simulink model "rtds_opal_aurora_synchronized"  (Simulink 10.0)
settings: Solver=ode4  StartTime=0.0  StopTime=inf  FixedStep=0.00005  RelTol=1e-3  EnableMultiTasking=on
PreLoadFcn:
  | Ts=50e-6;
InitFcn:
  | Ts=50e-6;
undefined symbols (not defined in the file): DUALSFP, EX, VC707_2
libraries: rtio_opalrt_common x8, rtlab x6, powerlib x6, simulink x3, xpcutilitieslib x1
Description:
  | Model of a simple control system for use iin training.
settings Model: Creator=Paul Baracos  LastModifiedBy=nei
settings Model: SuppressorTable=|
  | <?xml version="1.0" encoding="UTF-8" standalone="yes" ?>
  | <!DOCTYPE boost_serialization>
  | <boost_serialization signature="serialization::archive" version="15">
  | <DiagnosticSuppressor class_id="0" tracking_level="0" version="6">
  | 	<Table class_id="1" tracking_level="0" version="0">
  | 		<count>3</count>
  | 		<bucket_count>8</bucket_count>
  | 		<item_version>0</item_version>
  | 		<item class_id="2" tracking_level="0" version="0">
  | 			<first class_id="3" tracking_level="0" version="6">
  | 				<Source class_id="4" tracking_level="0" version="0">
  | 					<count>1</count>
  | 					<item_version>0</item_version>
  | 					<item>rtds_opal_aurora_synchronized/SM_Controller/Subsystem/Extract Bits</item>
  | 				</Source>
  | 			</first>
  | 			<second class_id="5" tracking_level="0" version="6">
  | 				<SuppressedData class_id="6" tracking_level="0" version="0">
  | 					<count>2</count>
  | 					<bucket_count>8</bucket_count>
  | 					<item_version>0</item_version>
  | 					<item class_id="7" tracking_level="0" version="0">
  | 						<first class_id="8" tracking_level="0" version="6">
  | 							<ID>Simulink:DataType:WarningOverFlowDetected</ID>
  | 							<Cause>
  | 								<Source>
  | 									<count>0</count>
  | 									<item_version>0</item_version>
  | 								</Source>
  | 							</Cause>
  | 						</first>
  | 						<second class_id="9" tracking_level="0" version="6">
  | 							<Comment></Comment>
  | 							<User></User>
  | 							<LastModified class_id="10" tracking_level="0" version="0">
  | 								<ptime_date class_id="11" tracking_level="0" version="0">
  | 									<date>20160608</date>
  | 								</ptime_date>
  | 								<ptime_time_duration class_id="12" tracking_level="0" version="0">
  | 									<is_special>0</is_special>
  | 									<time_duration_hours>15</time_duration_hours>
  | 									<time_duration_minutes>43</time_duration_minutes>
  | 									<time_duration_seconds>6</time_duration_seconds>
  | 									<time_duration_fractional_seconds>0</time_duration_fractional_seconds>
  | 								</ptime_time_duration>
  | 							</LastModified>
  | 							<SuppressionType>1</SuppressionType>
  | 						</second>
  | 					</item>
  | 					<item>
  | 						<first>
  | 							<ID>SimulinkFixedPoint:util:Overflowoccurred</ID>
  | 							<Cause>
  | 								<Source>
  | 									<count>0</count>
  | 									<item_version>0</item_version>
  | 								</Source>
  | 							</Cause>
  | 						</first>
  | 						<second>
  | 							<Comment></Comment>
  | 							<User></User>
  | 							<LastModified>
  | 								<ptime_date>
  | 									<date>20160608</date>
  | 								</ptime_date>
  | 								<ptime_time_duration>
  | 									<is_special>0</is_special>
  | 									<time_duration_hours>15</time_duration_hours>
  | 									<time_duration_minutes>43</time_duration_minutes>
  | 									<time_duration_seconds>6</time_duration_seconds>
  | 									<time_duration_fractional_seconds>0</time_duration_fractional_seconds>
  | 								</ptime_time_duration>
  | 							</LastModified>
  | 							<SuppressionType>1</SuppressionType>
  | 						</second>
  | 					</item>
  | 				</SuppressedData>
  | 			</second>
  | 		</item>
  | 		<item>
  | 			<first>
  | 				<Source>
  | 					<count>1</count>
  | 					<item_version>0</item_version>
  | 					<item>rtds_opal_aurora_synchronized/SM_Controller/Subsystem/Extract Bits1</item>
  | 				</Source>
  | 			</first>
  | 			<second>
  | 				<SuppressedData>
  | 					<count>2</count>
  | 					<bucket_count>8</bucket_count>
  | 					<item_version>0</item_version>
  | 					<item>
  | 						<first>
  | 							<ID>Simulink:DataType:WarningOverFlowDetected</ID>
  | 							<Cause>
  | 								<Source>
  | 									<count>0</count>
  | 									<item_version>0</item_version>
  | 								</Source>
  | 							</Cause>
  | 						</first>
  | 						<second>
  | 							<Comment></Comment>
  | 							<User></User>
  | 							<LastModified>
  | 								<ptime_date>
  | 									<date>20160608</date>
  | 								</ptime_date>
  | 								<ptime_time_duration>
  | 									<is_special>0</is_special>
  | 									<time_duration_hours>15</time_duration_hours>
  | 									<time_duration_minutes>43</time_duration_minutes>
  | 									<time_duration_seconds>6</time_duration_seconds>
  | 									<time_duration_fractional_seconds>0</time_duration_fractional_seconds>
  | 								</ptime_time_duration>
  | 							</LastModified>
  | 							<SuppressionType>1</SuppressionType>
  | 						</second>
  | 					</item>
  | 					<item>
  | 						<first>
  | 							<ID>SimulinkFixedPoint:util:Overflowoccurred</ID>
  | 							<Cause>
  | 								<Source>
  | 									<count>0</count>
  | 									<item_version>0</item_version>
  | 								</Source>
  | 							</Cause>
  | 						</first>
  | 						<second>
  | 							<Comment></Comment>
  | 							<User></User>
  | 							<LastModified>
  | 								<ptime_date>
  | 									<date>20160608</date>
  | 								</ptime_date>
  | 								<ptime_time_duration>
  | 									<is_special>0</is_special>
  | 									<time_duration_hours>15</time_duration_hours>
  | 									<time_duration_minutes>43</time_duration_minutes>
  | 									<time_duration_seconds>6</time_duration_seconds>
  | 									<time_duration_fractional_seconds>0</time_duration_fractional_seconds>
  | 								</ptime_time_duration>
  | 							</LastModified>
  | 							<SuppressionType>1</SuppressionType>
  | 						</second>
  | 					</item>
  | 				</SuppressedData>
  | 			</second>
  | 		</item>
  | 		<item>
  | 			<first>
  | 				<Source>
  | 					<count>1</count>
  | 					<item_version>0</item_version>
  | 					<item>rtds_opal_aurora_synchronized/SM_Controller/Subsystem/Counter Free-Running</item>
  | 				</Source>
  | 			</first>
  | 			<second>
  | 				<SuppressedData>
  | 					<count>2</count>
  | 					<bucket_count>8</bucket_count>
  | 					<item_version>0</item_version>
  | 					<item>
  | 						<first>
  | 							<ID>Simulink:DataType:WarningOverFlowDetected</ID>
  | 							<Cause>
  | 								<Source>
  | 									<count>0</count>
  | 									<item_version>0</item_version>
  | 								</Source>
  | 							</Cause>
  | 						</first>
  | 						<second>
  | 							<Comment></Comment>
  | 							<User></User>
  | 							<LastModified>
  | 								<ptime_date>
  | 									<date>20160523</date>
  | 								</ptime_date>
  | 								<ptime_time_duration>
  | 									<is_special>0</is_special>
  | 									<time_duration_hours>10</time_duration_hours>
  | 									<time_duration_minutes>57</time_duration_minutes>
  | 									<time_duration_seconds>55</time_duration_seconds>
  | 									<time_duration_fractional_seconds>0</time_duration_fractional_seconds>
  | 								</ptime_time_duration>
  | 							</LastModified>
  | 							<SuppressionType>1</SuppressionType>
  | 						</second>
  | 					</item>
  | 					<item>
  | 						<first>
  | 							<ID>SimulinkFixedPoint:util:Overflowoccurred</ID>
  | 							<Cause>
  | 								<Source>
  | 									<count>0</count>
  | 									<item_version>0</item_version>
  | 								</Source>
  | 							</Cause>
  | 						</first>
  | 						<second>
  | 							<Comment></Comment>
  | 							<User></User>
  | 							<LastModified>
  | 								<ptime_date>
  | 									<date>20160523</date>
  | 								</ptime_date>
  | 								<ptime_time_duration>
  | 									<is_special>0</is_special>
  | 									<time_duration_hours>10</time_duration_hours>
  | 									<time_duration_minutes>57</time_duration_minutes>
  | 									<time_duration_seconds>55</time_duration_seconds>
  | 									<time_duration_fractional_seconds>0</time_duration_fractional_seconds>
  | 								</ptime_time_duration>
  | 							</LastModified>
  | 							<SuppressionType>1</SuppressionType>
  | 						</second>
  | 					</item>
  | 				</SuppressedData>
  | 			</second>
  | 		</item>
  | 	</Table>
  | </DiagnosticSuppressor>
  | </boost_serialization>
settings DataIOCC: LimitDataPoints=on  SignalLoggingSaveFormat=ModelDataLogs  SaveOutput=off  SaveTime=off  SignalLoggingName=sigsOut
settings OptimizationCC: BlockReduction=off  BooleanDataType=off  OptimizeBlockIOStorage=off  BufferReuse=off  GlobalBufferReuse=off  ExpressionFolding=off  LocalBlockOutputs=off  InitFltsAndDblsToZero=on  OptimizeDataStoreBuffers=off  BusAssignmentInplaceUpdate=off
settings DebuggingCC: SaveWithParameterizedLinksMsg=none  SignalResolutionControl=TryResolveAllWithWarning  MultiTaskDSMMsg=warning  MultiTaskCondExecSysMsg=none  FcnCallInpInsideContextMsg=warning
settings HardwareCC: TargetUnknown=on
settings GRTTargetCC: TargetFcnLib=ansi_tfl_tmw.mat  GeneratePreprocessorConditionals=Disable all
settings ConfigComp: CovExternalEMLEnable=off

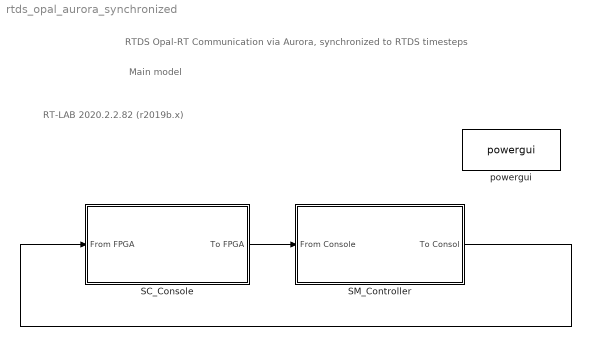
== system rtds_opal_aurora_synchronized ==
  note: Main model
  note: RT-LAB 2020.2.2.82 (r2019b.x)
  note: RTDS Opal-RT Communication via Aurora, synchronized to RTDS timesteps
  SC_Console : Subsystem
  SM_Controller : Subsystem
  powergui : powerlib/powergui  Priority=1  SimulationMode=Discrete  SampleTime=Ts  frequency=60  Iterations=50  frequencyindice=60  Pbase=100e6  ErrMax=1e-4  UnitsV=kV  UnitsW=MW  buscounter=0  FunctionMessages=off  echomessages=off  EnableUseOfTLC=off  CurrentSourceSwitches=off  DisableSnubberDevices=off  DisableRonSwitches=off  DisableVfSwitches=off  DisplayEquations=off  AutomaticDiscreteSolvers=off  SolverType=Backward Euler  Interpol=off  ExternalGateDelay=off  methode=off  Ts=0  x0status=blocks  SPID=off  SwTol=0  HookPort=off  NonlinearTolerance=1e-4  nMaxIteration=100  ContinueOnMaxIteration=off  RestoreLinks=warning  ResistiveCurrentMeasurement=off  Frange=[0:2:500]  Ylog=off  Xlog=on  ShowGrid=off  save=off  variable=ZData  structure=0  ZoomFFT=off  StartTime=0.0  cycles=1  DisplayStyle=1  fundamental=60  FreqAxis=off  MaxFrequency=1000  frequencyindicesteady=1  RmsSteady=1  display=off
      settings: SourceProductName=Simscape Electrical
  wires:
  SC_Console/1(To FPGA) -> SM_Controller/1(From Console)
  SM_Controller/1(To Consol) -> SC_Console/1(From FPGA)

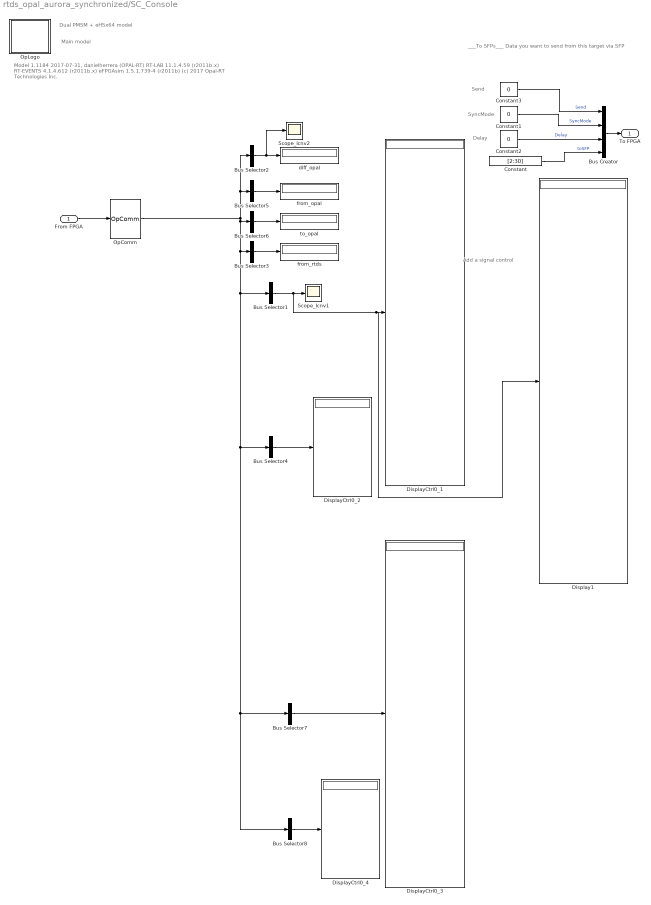
== system rtds_opal_aurora_synchronized/SC_Console ==
  note: Send
  note: Delay
  note: SyncMode
  note: Add a signal control
  note: ___To SFPs___
      | Data you want to send from this target via SFP
  note: Dual PMSM + eHSx64 model
  note: Main model
  note: Model                1.1184         2017-07-31, danielherrera (OPAL-RT)
      | RT-LAB            11.1.4.59    (r2011b.x)
      | RT-EVENTS    4.1.4.612      (r2011b.x)
      | eFPGAsim       1.5.1.739-4  (r2011b)
      | (c) 2017 Opal-RT Technologies Inc.
  From FPGA : Inport
  Bus Creator : BusCreator  Inputs=4
  Bus Selector1 : BusSelector  OutputSignals=SFP_RX_Data (signal 2)  OutputAsBus=on
  Bus Selector2 : BusSelector  OutputSignals=diff_opal (signal 3)  OutputAsBus=on
  Bus Selector3 : BusSelector  OutputSignals=from_rtds (signal 6)  OutputAsBus=on
  Bus Selector4 : BusSelector  OutputSignals=SFP_Status (signal 1)  OutputAsBus=on
  Bus Selector5 : BusSelector  OutputSignals=from_opal (signal 4)  OutputAsBus=on
  Bus Selector6 : BusSelector  OutputSignals=to_opal (signal 5)  OutputAsBus=on
  Bus Selector7 : BusSelector  OutputSignals=SFP_RX_Data (signal 8)  OutputAsBus=on
  Bus Selector8 : BusSelector  OutputSignals=SFP_Status (signal 7)  OutputAsBus=on
  Constant : Constant  Value=[2:30]
  Constant1 : Constant  Value=0  OutDataTypeStr=double
  Constant2 : Constant  Value=0  OutDataTypeStr=double
  Constant3 : Constant  Value=0  OutDataTypeStr=double
  Display1 : Display
  DisplayCtrl0_{1..4} (4 alike) : Display
  OpComm : rtlab/OpComm  nbport=1  groupe_acq=1  subsys_rate=0  st=0  Synchronization=on  Interpolation=on  Threshold=1.0  Missed_Data=off  Sim_Time=off  Samples=off  dynSigOut=off  from_console=0  warning_done=off  writeOpCommFile=off  Offset=off
      settings: SourceProductName=RT-LAB
  OpLogo : Subsystem
      mask Display:
      | opLogo = imread('efsOpLogo.tif','tif');
      | image(opLogo(:,:,1:3));
  Scope_Icnv1 : Scope
  Scope_Icnv2 : Scope
  diff_opal : Display
  from_opal : Display
  from_rtds : Display
  to_opal : Display
  To FPGA : Outport
  wires:
  From FPGA/1 -> OpComm/1
  Bus Selector1/1 -> Display1/1, DisplayCtrl0_1/1, Scope_Icnv1/1
  Bus Selector4/1 -> DisplayCtrl0_2/1
  Bus Creator/1 -> To FPGA/1
  Constant1/1 -> Bus Creator/2  "SyncMode"
  Constant/1 -> Bus Creator/4  "toSFP"
  Constant2/1 -> Bus Creator/3  "Delay"
  Constant3/1 -> Bus Creator/1  "Send"
  Bus Selector2/1 -> Scope_Icnv2/1, diff_opal/1
  Bus Selector3/1 -> from_rtds/1
  Bus Selector5/1 -> from_opal/1
  Bus Selector6/1 -> to_opal/1
  OpComm/1 -> Bus Selector5/1, Bus Selector2/1, Bus Selector6/1, Bus Selector8/1, Bus Selector7/1, Bus Selector4/1, Bus Selector1/1, Bus Selector3/1
  Bus Selector8/1 -> DisplayCtrl0_4/1
  Bus Selector7/1 -> DisplayCtrl0_3/1

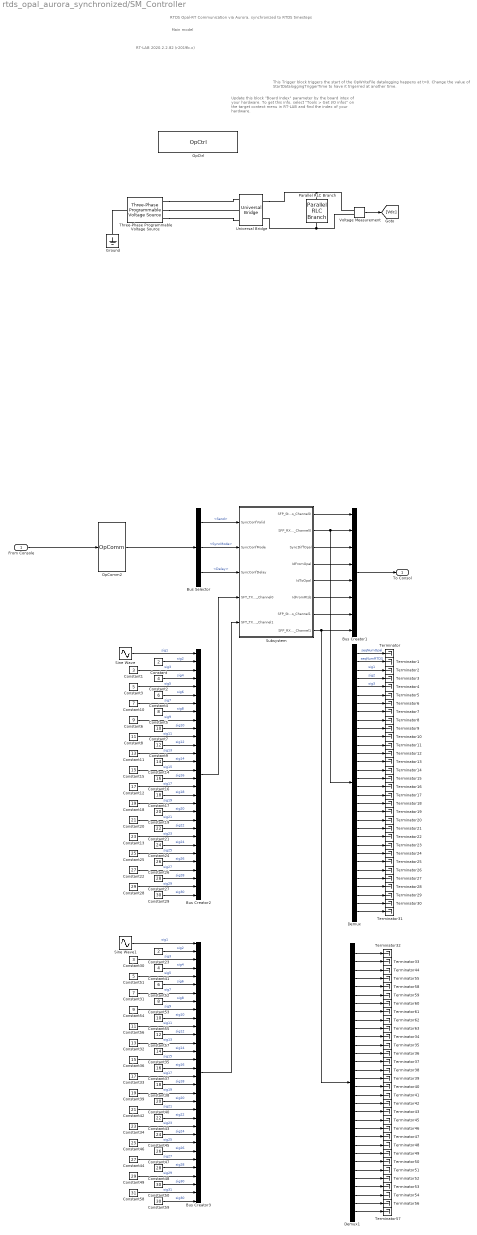
== system rtds_opal_aurora_synchronized/SM_Controller ==
  note: Update this block "Board Index" parameter by the
      | board intex of your hardware. To get this info, select
      | "Tools > Get I/O infos" on the target context menu
      | in RT-LAB and find the index of your hardware.
  note: This Trigger block triggers the start of the OpWriteFile datalogging happens at t=0. Change the value of StartDataloggingTriggerTime to have it trigerred at another time.
  note: Main model
  note: RTDS Opal-RT Communication via Aurora, synchronized to RTDS timesteps
  note: RT-LAB 2020.2.2.82 (r2019b.x)
  From Console : Inport
  Bus Selector : BusSelector  OutputSignals=Send,SyncMode,Delay
  Bus Creator1 : BusCreator  Inputs=8
  Bus Creator2 : BusCreator  Inputs=30
  Bus Creator3 : BusCreator  Inputs=32
  Constant : Constant  Value=2
  Constant1 : Constant  Value=3
  Constant10 : Constant  Value=7
  Constant11 : Constant  Value=13
  Constant12 : Constant  Value=17
  Constant13 : Constant  Value=23
  Constant14 : Constant  Value=14
  Constant15 : Constant  Value=15
  Constant16 : Constant  Value=16
  Constant17 : Constant  Value=18
  Constant18 : Constant  Value=19
  Constant19 : Constant  Value=20
  Constant2 : Constant  Value=4
  Constant20 : Constant  Value=21
  Constant21 : Constant  Value=22
  Constant22 : Constant  Value=27
  Constant23 : Constant  Value=2
  Constant24 : Constant  Value=24
  Constant25 : Constant  Value=25
  Constant26 : Constant  Value=26
  Constant27 : Constant  Value=28
  Constant28 : Constant  Value=29
  Constant29 : Constant  Value=30
  Constant3 : Constant  Value=5
  Constant30 : Constant  Value=3
  Constant31 : Constant  Value=7
  Constant32 : Constant  Value=13
  Constant33 : Constant  Value=17
  Constant34 : Constant  Value=23
  Constant35 : Constant  Value=14
  Constant36 : Constant  Value=15
  Constant37 : Constant  Value=16
  Constant38 : Constant  Value=18
  Constant39 : Constant  Value=19
  Constant4 : Constant  Value=6
  Constant40 : Constant  Value=20
  Constant41 : Constant  Value=4
  Constant42 : Constant  Value=21
  Constant43 : Constant  Value=22
  Constant44 : Constant  Value=27
  Constant45 : Constant  Value=24
  Constant46 : Constant  Value=25
  Constant47 : Constant  Value=26
  Constant48 : Constant  Value=28
  Constant49 : Constant  Value=29
  Constant5 : Constant  Value=8
  Constant50 : Constant  Value=30
  Constant51 : Constant  Value=5
  Constant52 : Constant  Value=6
  Constant53 : Constant  Value=8
  Constant54 : Constant  Value=9
  Constant55 : Constant  Value=10
  Constant56 : Constant  Value=11
  Constant57 : Constant  Value=12
  Constant58 : Constant  Value=31
  Constant59 : Constant  Value=30
  Constant6 : Constant  Value=9
  Constant7 : Constant  Value=10
  Constant8 : Constant  Value=11
  Constant9 : Constant  Value=12
  Demux : Demux  Outputs=32
  Demux1 : Demux  Outputs=32
  Ground : powerlib/Elements/Ground  LConnTagsString=a
      settings: SourceProductName=Simscape Electrical
  OpComm2 : rtlab/OpComm  nbport=1  groupe_acq=1  subsys_rate=Ts  st=0  Synchronization=on  Interpolation=on  Threshold=1.0  Missed_Data=off  Sim_Time=off  Samples=off  dynSigOut=off  from_console=1  warning_done=off  writeOpCommFile=off  Offset=off
      settings: SourceProductName=RT-LAB
  OpCtrl : rtio_opalrt_common/OpCtrl  CtrlName='OpCtrl'  boardid=0  BitstreamFilename=D:\OPAL-RT\RT-LABv2020_Workspace\aurora_cpu_ch0_rtxsg\VC707_2-EX-0001-3_2_10_45-DUALSFP-02-24  numconfig=-1  mode=Master with external clock  externalClock=off  decimRtsi=0  calibIO=off  SampleTime=0  loadinport=-1  BoardType=VC707  SecondaryPresent=off  sync_type=Optical fiber  scope_enable=off  fsdFileName=VC707_2-EX-0001-3_2_10_45-DUALSFP-02-24.fsd
  Parallel RLC Branch : powerlib/Elements/Parallel RLC Branch  LConnTagsString=a  RConnTagsString=__new0  BranchType=RC  Resistance=100  Inductance=1e-3  SetiL0=off  InitialCurrent=0  Capacitance=10e-3  Setx0=off  InitialVoltage=0  Measurements=None
      settings: SourceProductName=Simscape Electrical
  Sine Wave : Sin  Amplitude=10  Frequency=50*pi*2  SampleTime=0
  Sine Wave1 : Sin  Amplitude=10  Frequency=50*pi*2  SampleTime=0
  Subsystem : Subsystem
  Terminator{,1..63} (64 alike) : Terminator
  Three-Phase Programmable Voltage Source : powerlib/Electrical Sources/Three-Phase Programmable Voltage Source  PositiveSequence="[90  0 60]"  VariationEntity=None  VariationType=Table of time-amplitude pairs  VariationTypeAlt=Step  VariationStep=0.5  VariationRate=10  VariationMagnitude=0.3  VariationFrequency=2  VariationTiming=[1 2]  VariationPhaseA=off  Amplitudes=[1 0.8 1.2 1.0]  TimeValues=[0 0.1 0.15 0.2]  HarmonicGeneration=off  HarmonicA=[3 0.2 -25 0]  HarmonicB=[2 0.15 35 2]  Timing="[0.05  3]"  BusType=swing  Pref=0  Qref=0  Qmin=-inf  Qmax=inf
      settings: SourceProductName=Simscape Electrical
  Universal Bridge : powerlib/Power Electronics/Universal Bridge  Arms=3  SnubberResistance=1e5  SnubberCapacitance=inf  Device=Diodes  Ron=1e-3  Lon=0  ForwardVoltages="[  0  0  ]"  ForwardVoltage=0  GTOparameters=[ 10e-6 , 20e-6 ]  IGBTparameters=[ 1e-6 , 2e-6 ]  Measurements=None  Measurements_2=None  converterType=Rectifier
      settings: SourceProductName=Simscape Electrical
  Voltage Measurement : powerlib/Measurements/Voltage Measurement  PhasorSimulation=off  OutputType=Complex  PSBequivalent=0
      settings: SourceProductName=Simscape Electrical
  To Consol : Outport
  wires:
  Voltage Measurement/1 -> [Vdc]
  Bus Creator1/1 -> To Consol/1
  From Console/1 -> OpComm2/1
  OpComm2/1 -> Bus Selector/1
  Bus Selector/1 -> Subsystem/1(SyncConfValid)  "<Send>"
  Bus Selector/2 -> Subsystem/2(SyncConfMode)  "<SyncMode>"
  Bus Selector/3 -> Subsystem/3(SyncConfDelay)  "<Delay>"
  Subsystem/1(SFP_Status_Channel0) -> Bus Creator1/1
  Subsystem/2(SFP_RX_Data_Channel0) -> Demux/1, Bus Creator1/2
  Subsystem/3(SyncDiffOpal) -> Bus Creator1/3
  Subsystem/4(IdFromOpal) -> Bus Creator1/4
  Subsystem/5(IdToOpal) -> Bus Creator1/5
  Subsystem/6(IdFromRtds) -> Bus Creator1/6
  Bus Creator2/1 -> Subsystem/4(SFT_TX_Data_Channel0)
  Sine Wave/1 -> Bus Creator2/1  "sig1"
  Constant/1 -> Bus Creator2/2  "sig2"
  Constant1/1 -> Bus Creator2/3  "sig3"
  Constant2/1 -> Bus Creator2/4  "sig4"
  Constant4/1 -> Bus Creator2/6  "sig6"
  Constant3/1 -> Bus Creator2/5  "sig5"
  Constant5/1 -> Bus Creator2/8  "sig8"
  Constant7/1 -> Bus Creator2/10  "sig10"
  Constant8/1 -> Bus Creator2/11  "sig11"
  Constant6/1 -> Bus Creator2/9  "sig9"
  Constant9/1 -> Bus Creator2/12  "sig12"
  Constant10/1 -> Bus Creator2/7  "sig7"
  Constant11/1 -> Bus Creator2/13  "sig13"
  Constant14/1 -> Bus Creator2/14  "sig14"
  Constant21/1 -> Bus Creator2/22  "sig22"
  Constant12/1 -> Bus Creator2/17  "sig17"
  Constant20/1 -> Bus Creator2/21  "sig21"
  Constant18/1 -> Bus Creator2/19  "sig19"
  Constant15/1 -> Bus Creator2/15  "sig15"
  Constant16/1 -> Bus Creator2/16  "sig16"
  Constant19/1 -> Bus Creator2/20  "sig20"
  Constant17/1 -> Bus Creator2/18  "sig18"
  Constant13/1 -> Bus Creator2/23  "sig23"
  Constant26/1 -> Bus Creator2/26  "sig26"
  Constant25/1 -> Bus Creator2/25  "sig25"
  Constant24/1 -> Bus Creator2/24  "sig24"
  Constant28/1 -> Bus Creator2/29  "sig29"
  Constant27/1 -> Bus Creator2/28  "sig28"
  Constant22/1 -> Bus Creator2/27  "sig27"
  Demux/1 -> Terminator/1  "seqNumOpal"
  Demux/2 -> Terminator1/1  "seqNumRTDS"
  Demux/4 -> Terminator3/1  "sig2"
  Demux/3 -> Terminator2/1  "sig1"
  Demux/8 -> Terminator7/1
  Demux/7 -> Terminator6/1
  Demux/6 -> Terminator5/1
  Demux/5 -> Terminator4/1  "sig3"
  Demux/9 -> Terminator8/1
  Demux/15 -> Terminator14/1
  Demux/10 -> Terminator9/1
  Demux/14 -> Terminator13/1
  Demux/13 -> Terminator12/1
  Demux/12 -> Terminator11/1
  Demux/16 -> Terminator15/1
  Demux/11 -> Terminator10/1
  Demux/17 -> Terminator16/1
  Demux/23 -> Terminator22/1
  Demux/18 -> Terminator17/1
  Demux/22 -> Terminator21/1
  Demux/21 -> Terminator20/1
  Demux/20 -> Terminator19/1
  Demux/24 -> Terminator23/1
  Demux/19 -> Terminator18/1
  Demux/25 -> Terminator24/1
  Demux/31 -> Terminator30/1
  Demux/26 -> Terminator25/1
  Demux/30 -> Terminator29/1
  Demux/29 -> Terminator28/1
  Demux/28 -> Terminator27/1
  Demux/32 -> Terminator31/1
  Demux/27 -> Terminator26/1
  Constant48/1 -> Bus Creator3/28  "sig28"
  Constant39/1 -> Bus Creator3/19  "sig19"
  Constant32/1 -> Bus Creator3/13  "sig13"
  Constant38/1 -> Bus Creator3/18  "sig18"
  Constant30/1 -> Bus Creator3/3  "sig3"
  Constant40/1 -> Bus Creator3/20  "sig20"
  Constant41/1 -> Bus Creator3/4  "sig4"
  Constant52/1 -> Bus Creator3/6  "sig6"
  Constant44/1 -> Bus Creator3/27  "sig27"
  Constant34/1 -> Bus Creator3/23  "sig23"
  Constant50/1 -> Bus Creator3/30  "sig30"
  Constant45/1 -> Bus Creator3/24  "sig24"
  Constant47/1 -> Bus Creator3/26  "sig26"
  Constant46/1 -> Bus Creator3/25  "sig25"
  Constant33/1 -> Bus Creator3/17  "sig17"
  Constant31/1 -> Bus Creator3/7  "sig7"
  Constant56/1 -> Bus Creator3/11  "sig11"
  Constant51/1 -> Bus Creator3/5  "sig5"
  Constant37/1 -> Bus Creator3/16  "sig16"
  Constant57/1 -> Bus Creator3/12  "sig12"
  Constant35/1 -> Bus Creator3/14  "sig14"
  Constant23/1 -> Bus Creator3/2  "sig2"
  Constant42/1 -> Bus Creator3/21  "sig21"
  Constant54/1 -> Bus Creator3/9  "sig9"
  Constant53/1 -> Bus Creator3/8  "sig8"
  Sine Wave1/1 -> Bus Creator3/1  "sig1"
  Constant55/1 -> Bus Creator3/10  "sig10"
  Constant36/1 -> Bus Creator3/15  "sig15"
  Constant43/1 -> Bus Creator3/22  "sig22"
  Constant49/1 -> Bus Creator3/29  "sig29"
  Bus Creator3/1 -> Subsystem/5(SFT_TX_Data_Channel1)
  Demux1/27 -> Terminator51/1
  Demux1/32 -> Terminator57/1
  Demux1/2 -> Terminator33/1
  Demux1/25 -> Terminator49/1
  Demux1/17 -> Terminator40/1
  Demux1/8 -> Terminator61/1
  Demux1/7 -> Terminator60/1
  Demux1/14 -> Terminator37/1
  Demux1/30 -> Terminator54/1
  Demux1/22 -> Terminator46/1
  Demux1/31 -> Terminator56/1
  Demux1/26 -> Terminator50/1
  Demux1/19 -> Terminator42/1
  Demux1/28 -> Terminator52/1
  Demux1/4 -> Terminator55/1
  Demux1/15 -> Terminator38/1
  Demux1/12 -> Terminator35/1
  Demux1/23 -> Terminator47/1
  Demux1/21 -> Terminator45/1
  Demux1/29 -> Terminator53/1
  Demux1/11 -> Terminator34/1
  Demux1/16 -> Terminator39/1
  Demux1/10 -> Terminator63/1
  Demux1/24 -> Terminator48/1
  Demux1/20 -> Terminator43/1
  Demux1/1 -> Terminator32/1
  Demux1/13 -> Terminator36/1
  Demux1/6 -> Terminator59/1
  Demux1/18 -> Terminator41/1
  Demux1/9 -> Terminator62/1
  Demux1/5 -> Terminator58/1
  Demux1/3 -> Terminator44/1
  Subsystem/8(SFP_RX_Data_Channel1) -> Bus Creator1/8, Demux1/1
  Subsystem/7(SFP_Status_Channel1) -> Bus Creator1/7
  Constant59/1 -> Bus Creator3/32  "sig30"
  Constant58/1 -> Bus Creator3/31  "sig31"
  Constant29/1 -> Bus Creator2/30  "sig30"
  connections:
  Parallel RLC Branch/LConn1 -- Universal Bridge/RConn1 -- Voltage Measurement/LConn1
  Voltage Measurement/LConn2 -- Parallel RLC Branch/RConn1 -- Universal Bridge/RConn2
  Three-Phase Programmable Voltage Source/RConn1 -- Universal Bridge/LConn1
  Three-Phase Programmable Voltage Source/RConn3 -- Universal Bridge/LConn3
  Three-Phase Programmable Voltage Source/RConn2 -- Universal Bridge/LConn2
  Ground/LConn1 -- Three-Phase Programmable Voltage Source/LConn1

== system rtds_opal_aurora_synchronized/SC_Console/OpLogo ==

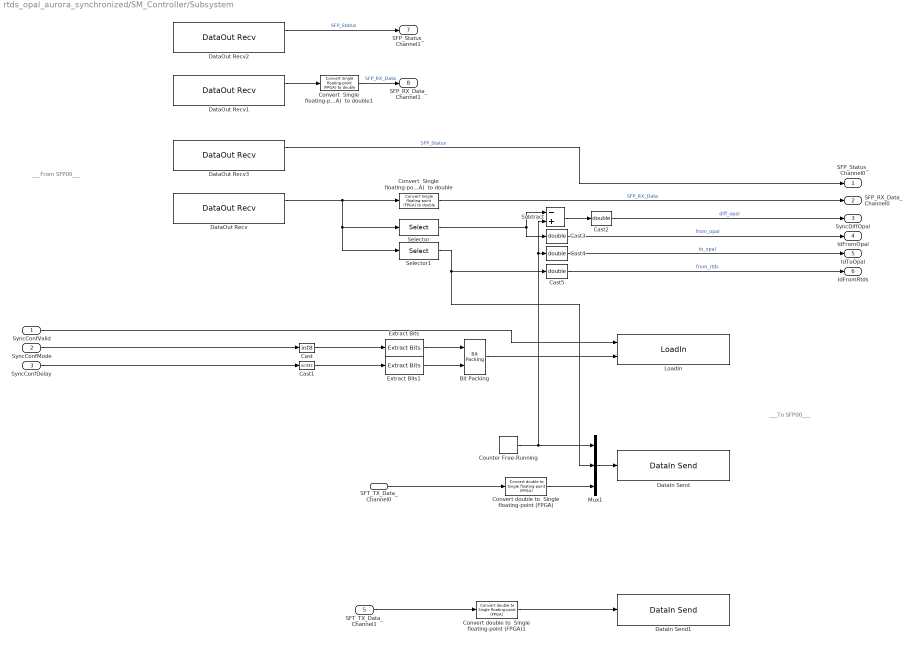
== system rtds_opal_aurora_synchronized/SM_Controller/Subsystem ==
  note: ___To SFP00___
  note: ___From SFP00___
  SyncConfValid : Inport
  SyncConfMode : Inport  Port=2
  SyncConfDelay : Inport  Port=3
  SFT_TX_Data_Channel0 : Inport  Port=4
  SFT_TX_Data_Channel1 : Inport  Port=5
  "Bit Packing " : xpcutilitieslib/Bit Packing   MaskBitPatterns={[0:2] [3:22]}  MaskPackDataType=uint32  MaskPackDataSize=[1]
      settings: SourceProductName=Simulink Real-Time  SourceProductBaseCode=XP
  Cast : DataTypeConversion  OutDataTypeStr=int8
  Cast1 : DataTypeConversion  OutDataTypeStr=uint32
  Cast{2..5} (4 alike) : DataTypeConversion  OutDataTypeStr=double
  Convert  Single floating-point (FPGA)  to double : rtlab/Miscellaneous/Convert  Single floating-point (FPGA)  to double
      settings: SourceProductName=RT-LAB
  Convert  Single floating-point (FPGA)  to double1 : rtlab/Miscellaneous/Convert  Single floating-point (FPGA)  to double
      settings: SourceProductName=RT-LAB
  Convert double to  Single floating-point (FPGA) : rtlab/Miscellaneous/Convert double to  Single floating-point (FPGA)
      settings: SourceProductName=RT-LAB
  Convert double to  Single floating-point (FPGA)1 : rtlab/Miscellaneous/Convert double to  Single floating-point (FPGA)
      settings: SourceProductName=RT-LAB
  Counter Free-Running : simulink/Sources/Counter Free-Running  NumBits=32  tsamp=Ts
  DataIn Send : rtio_opalrt_common/DataIn Send  CtrlName='OpCtrl'  FcnNos=1  width=32  portType=uint32  checkVersion=off  expectedId=0  expectedVersion=0  opComp=>=
      settings: AttributesFormatString=%<CtrlName>
  DataIn Send1 : rtio_opalrt_common/DataIn Send  CtrlName='OpCtrl'  FcnNos=2  width=32  portType=uint32  checkVersion=off  expectedId=0  expectedVersion=0  opComp=>=
      settings: AttributesFormatString=%<CtrlName>
  DataOut Recv : rtio_opalrt_common/DataOut Recv  CtrlName='OpCtrl'  FcnNos=1  width=32  portType=uint32  sampleTime=0  checkVersion=off  expectedId=0  expectedVersion=0  opComp=>=
      settings: AttributesFormatString=%<CtrlName>
  DataOut Recv1 : rtio_opalrt_common/DataOut Recv  CtrlName='OpCtrl'  FcnNos=3  width=32  portType=uint32  sampleTime=0  checkVersion=off  expectedId=0  expectedVersion=0  opComp=>=
      settings: AttributesFormatString=%<CtrlName>
  DataOut Recv2 : rtio_opalrt_common/DataOut Recv  CtrlName='OpCtrl'  FcnNos=4  width=5  portType=double  sampleTime=0  checkVersion=off  expectedId=0  expectedVersion=0  opComp=>=
      settings: AttributesFormatString=%<CtrlName>
  DataOut Recv3 : rtio_opalrt_common/DataOut Recv  CtrlName='OpCtrl'  FcnNos=2  width=5  portType=double  sampleTime=0  checkVersion=off  expectedId=0  expectedVersion=0  opComp=>=
      settings: AttributesFormatString=%<CtrlName>
  Extract Bits : simulink/Logic and Bit Operations/Extract Bits  bitsToExtract=Range ending with least significant bit  numBits=3  bitIdxRange=[0 7]  outScalingMode=Treat bit field as an integer
      settings: SourceProductName=Simulink
  Extract Bits1 : simulink/Logic and Bit Operations/Extract Bits  bitsToExtract=Range ending with least significant bit  numBits=20  bitIdxRange=[0 7]  outScalingMode=Treat bit field as an integer
      settings: SourceProductName=Simulink
  LoadIn : rtio_opalrt_common/LoadIn  CtrlName='OpCtrl'  FcnNos=1  width=1  portType=uint32
      settings: AttributesFormatString=%<CtrlName>
  Mux1 : Mux  Inputs=3
  Selector : Selector  InputPortWidth=32  IndexOptions=Index vector (dialog)  Indices=[1]  OutputSizes=1
  Selector1 : Selector  InputPortWidth=32  IndexOptions=Index vector (dialog)  Indices=[32]  OutputSizes=1
  Subtract : Sum  Inputs=-+
  SFP_Status_Channel0 : Outport
  SFP_RX_Data_Channel0 : Outport  Port=2
  SyncDiffOpal : Outport  Port=3
  IdFromOpal : Outport  Port=4
  IdToOpal : Outport  Port=5
  IdFromRtds : Outport  Port=6
  SFP_Status_Channel1 : Outport  Port=7
  SFP_RX_Data_Channel1 : Outport  Port=8
  wires:
  Cast/1 -> Extract Bits/1
  Selector/1 -> Subtract/1, Cast3/1
  Subtract/1 -> Cast2/1
  DataOut Recv3/1 -> SFP_Status_Channel0/1  "SFP_Status"
  Mux1/1 -> DataIn Send/1
  Extract Bits1/1 -> "Bit Packing "/2
  DataOut Recv/1 -> Selector1/1, Selector/1, Convert  Single floating-point (FPGA)  to double/1
  Convert double to  Single floating-point (FPGA)/1 -> Mux1/3
  Extract Bits/1 -> "Bit Packing "/1
  Counter Free-Running/1 -> Mux1/1, Cast4/1, Subtract/2
  "Bit Packing "/1 -> LoadIn/2
  Cast5/1 -> IdFromRtds/1  "from_rtds"
  Cast1/1 -> Extract Bits1/1
  SFT_TX_Data_Channel0/1 -> Convert double to  Single floating-point (FPGA)/1
  Cast3/1 -> IdFromOpal/1  "from_opal"
  Cast4/1 -> IdToOpal/1  "to_opal"
  Cast2/1 -> SyncDiffOpal/1  "diff_opal"
  SyncConfMode/1 -> Cast/1
  SyncConfValid/1 -> LoadIn/1
  SyncConfDelay/1 -> Cast1/1
  Convert  Single floating-point (FPGA)  to double/1 -> SFP_RX_Data_Channel0/1  "SFP_RX_Data"
  SFT_TX_Data_Channel1/1 -> Convert double to  Single floating-point (FPGA)1/1
  Convert double to  Single floating-point (FPGA)1/1 -> DataIn Send1/1
  DataOut Recv1/1 -> Convert  Single floating-point (FPGA)  to double1/1
  Convert  Single floating-point (FPGA)  to double1/1 -> SFP_RX_Data_Channel1/1  "SFP_RX_Data"
  DataOut Recv2/1 -> SFP_Status_Channel1/1  "SFP_Status"
  Selector1/1 -> Cast5/1, Mux1/2
